simulink model "Lab44"  (R2020b)
settings: Solver=VariableStepAuto  StartTime=0.0  StopTime=10.0  RelTol=1e-3
settings Model: Creator=evpet  LastModifiedBy=evpet

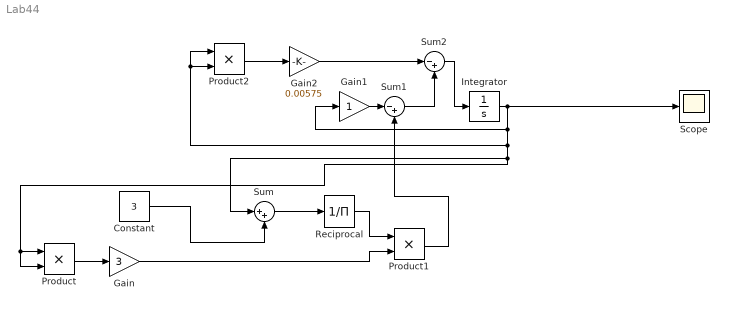
== system Lab44 ==
  Constant : Constant  Value=3
  Gain : Gain  Gain=3
  Gain1 : Gain
  Gain2 : Gain  Gain=0.00575
  Integrator : Integrator  InitialCondition=10
  Product : Product
  Product1 : Product
  Product2 : Product
  Reciprocal : Product  Inputs=/
  Scope : Scope
  Sum : Sum  Inputs=|++
  Sum1 : Sum  Inputs=|-+
  Sum2 : Sum  Inputs=|-+
  wires:
  Gain/1 -> Product1/2
  Product/1 -> Gain/1
  Reciprocal/1 -> Product1/1
  Constant/1 -> Sum/2
  Sum/1 -> Reciprocal/1
  Gain1/1 -> Sum1/1
  Integrator/1 -> Product2/2, Product2/1, Sum/1, Product/1, Product/2, Gain1/1, Scope/1
  Product1/1 -> Sum1/2
  Sum1/1 -> Sum2/2
  Product2/1 -> Gain2/1
  Gain2/1 -> Sum2/1
  Sum2/1 -> Integrator/1
